simulink model "model1_dyskretny"  (R2019b)
settings: Solver=FixedStepAuto  StartTime=0.0  StopTime=30  FixedStep=1  RelTol=1e-3
settings Model: Creator=dominik  LastModifiedBy=a.kuligowski
settings DataIOCC: ReturnWorkspaceOutputs=off
settings DebuggingCC: ArithmeticOperatorsInVariantConditions=warning
settings SFSimCC: SimUseLocalCustomCode=off  CustomCodeUndefinedFunction=UseInterfaceOnly
settings RTWCC: RTWUseLocalCustomCode=off

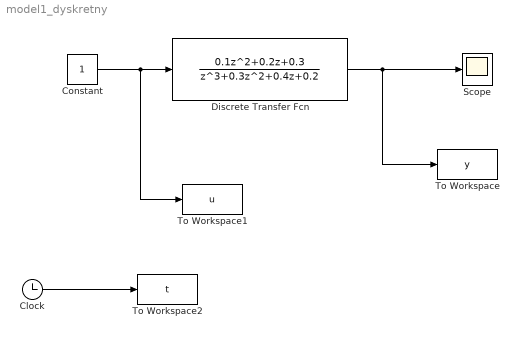
== system model1_dyskretny ==
  Clock : Clock
  Constant : Constant
  Discrete Transfer Fcn : DiscreteTransferFcn  Numerator=[0.1 0.2 0.3]  Denominator=[1 +0.3 0.4 0.2]  SampleTime=1
  Scope : Scope
  To Workspace : ToWorkspace  VariableName=y  SampleTime=-1
  To Workspace1 : ToWorkspace  VariableName=u  SampleTime=-1
  To Workspace2 : ToWorkspace  VariableName=t  SampleTime=-1
  wires:
  Constant/1 -> To Workspace1/1, Discrete Transfer Fcn/1
  Discrete Transfer Fcn/1 -> To Workspace/1, Scope/1
  Clock/1 -> To Workspace2/1
